simulink model "hcm_segway"  (R2017b)
settings: Solver=ode8  StartTime=0.0  StopTime=10  FixedStep=time_step/10  RelTol=1e-3
values from neighbouring files (symbols this model uses):
  front_rear = 0    [init.m]
  setV = 0    [init.m]
  your_dut = 18    [init.m]
undefined symbols (not defined in the file or in its folder): hcm, sigbuilder_block, Zs0, Zu0
libraries: simulink x2
settings Model: Creator=rvorster  LastModifiedBy=rvorster
settings CodeAppCC: StateflowObjectComments=on
settings SimscapeCC: SimscapeNormalizeSystem=off

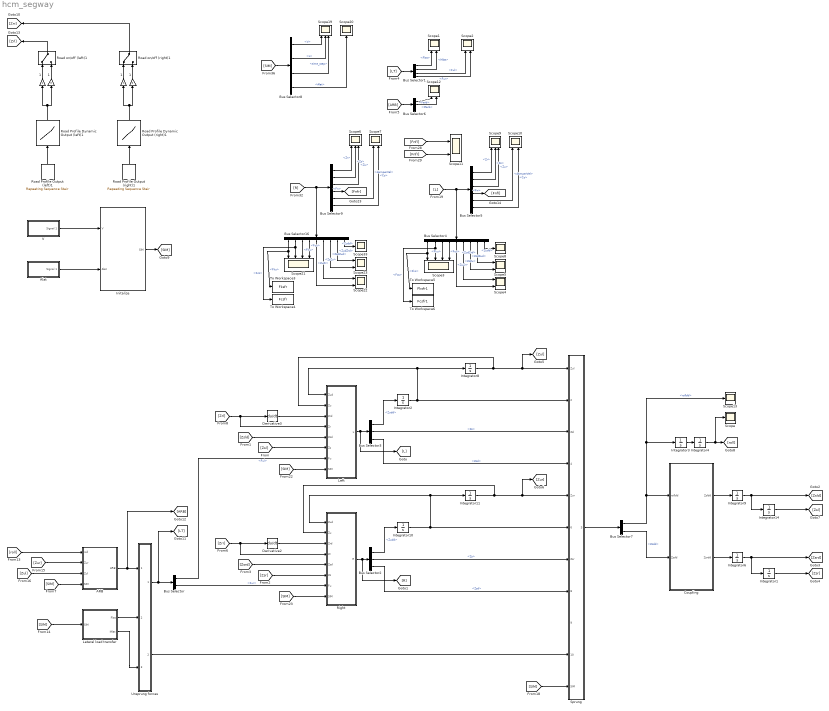
== system hcm_segway ==
  " 1" : Gain  Gain=0
  " 1" : Gain  Gain=0
  " 1" : Gain
  " 1" : Gain
  "ARB " : MATLAB Function  TreatAsAtomicUnit=on
  Alat : Subsystem  Tag=STV Subsys  LoadFcn=sigbuilder_block('load');  StartFcn=sigbuilder_block('start');  StopFcn=sigbuilder_block('stop');  ClipboardFcn=sigbuilder_block('clipboard');  mask(Sigbuilder block){tuvar=[0:10]}
      mask help: Simulink:masks:SigbuilderBlock_MD
      mask init:
      | if ~strcmp(get_param(bdroot(gcbh),'SimulationStatus'),'stopped') tuvar = sigbuilder_block('maskInit'); end
      settings: CopyFcn=sigbuilder_block('copy');  DeleteFcn=sigbuilder_block('delete');  ModelCloseFcn=sigbuilder_block('modelClose');  PreSaveFcn=sigbuilder_block('preSave');  PauseFcn=sigbuilder_block('pause');  ContinueFcn=sigbuilder_block('continue');  NameChangeFcn=sigbuilder_block('namechange');  OpenFcn=sigbuilder_block('open',[429.75 192 565.5 402.75 ]);  CloseFcn=sigbuilder_block('close');
      mask Display: plot(0, 0, 100, 100,[2, 2, 32, 32, 2], [68, 8, 8, 68, 68],[32, 2], [38, 38], [32, 19, 2],[53, 60, 44], [32, 17, 17, 2],[16, 16, 31, 31]);txt = getActiveGroup(gcbh);text(2, 100, txt,'verticalAlignment', 'top');
  Bus Selector : BusSelector  OutputSignals=Ful,Fur
  Bus Selector1 : BusSelector  OutputSignals=Flat,Mlat,Ful,Fur
  Bus Selector16 : BusSelector  OutputSignals=Fks,Fcs,Fku,Fcu,ZuZr,ZsZu,ZsdZud,ZudZrd,Zudd
  Bus Selector2 : BusSelector  OutputSignals=Zudd,Zs,Zsd
  Bus Selector3 : BusSelector  OutputSignals=Zudd,Zs,Zsd
  Bus Selector4 : BusSelector  OutputSignals=Fks,Fcs,Fku,Fcu,ZuZr,ZsZu,ZsdZud,ZudZrd,Zudd
  Bus Selector5 : BusSelector  OutputSignals=Zr,Zs,Zu,Fn,damperVel,Cs
  Bus Selector6 : BusSelector  OutputSignals=Farb,Marb,roll_u
  Bus Selector7 : BusSelector  OutputSignals=rolldd,Zsdd
  Bus Selector8 : BusSelector  OutputSignals=V,L,time_step,Alat
  Bus Selector9 : BusSelector  OutputSignals=Zr,Zs,Zu,Fn,damperVel,Cs
  Coupling : MATLAB Function  TreatAsAtomicUnit=on
  Derivative2 : Derivative
  Derivative3 : Derivative
  Initalize : MATLAB Function  TreatAsAtomicUnit=on
  Integrator1 : Integrator  InitialCondition=-Zs0(2)
  Integrator{2..4,6,9..10} (6 alike) : Integrator
  Integrator11 : Integrator  InitialCondition=-Zu0(2)
  Integrator14 : Integrator  InitialCondition=-Zs0(1)
  Integrator8 : Integrator  InitialCondition=-Zu0(1)
  Lateral load transfer : MATLAB Function  TreatAsAtomicUnit=on
  Left : MATLAB Function  TreatAsAtomicUnit=on
  Right : MATLAB Function  TreatAsAtomicUnit=on
  Road Profile Dynamic Output (left)1 : Lookup_n-D  NumberOfTableDimensions=1  BreakpointsForDimension1=[-5:5]  Table=tanh([-5:5])  InternalRulePriority=Speed  RndMeth=Simplest  InputSameDT=on
  Road Profile Dynamic Output (right)1 : Lookup_n-D  NumberOfTableDimensions=1  BreakpointsForDimension1=[-5:5]  Table=tanh([-5:5])  InternalRulePriority=Speed  RndMeth=Simplest  InputSameDT=on
  Road Profile Output (left)1 : simulink/Sources/Repeating Sequence Stair  OutValues=hx_left  tsamp=time_step  OutMin=[]  OutMax=[]  OutDataTypeStr=double  OutputDataTypeScalingMode=double  OutDataType=fixdt(0,8)  ConRadixGroup=Best Precision: Vector-wise  OutScaling=2^-12
  Road Profile Output (right)1 : simulink/Sources/Repeating Sequence Stair  OutValues=hx_right  tsamp=time_step  OutMin=[]  OutMax=[]  OutDataTypeStr=double  OutputDataTypeScalingMode=double  OutDataType=fixdt(0,8)  ConRadixGroup=Best Precision: Vector-wise  OutScaling=2^-12
  Road on/off (left)1 : ManualSwitch
  Road on/off (right)1 : ManualSwitch
  Scope{,8,13,20,33} (5 alike) : Scope
  Scope{1..2,4..5,7,10..12,22..23} (10 alike) : Scope  NumInputPorts=2
  Scope19 : Scope  NumInputPorts=3
  Scope21 : Scope  NumInputPorts=4
  Scope3 : Scope  NumInputPorts=4
  Scope6 : Scope  NumInputPorts=3
  Scope9 : Scope  NumInputPorts=3
  Sprung : MATLAB Function  TreatAsAtomicUnit=on
  To Workspace3 : ToWorkspace  VariableName=Fksfr  SaveFormat=Timeseries  SampleTime=-1
  To Workspace4 : ToWorkspace  VariableName=Fcsfr  SaveFormat=Timeseries  SampleTime=-1
  To Workspace5 : ToWorkspace  VariableName=Fksfr1  SaveFormat=Timeseries  SampleTime=-1
  To Workspace6 : ToWorkspace  VariableName=Fcsfr1  SaveFormat=Timeseries  SampleTime=-1
  Unsprung forces : MATLAB Function  TreatAsAtomicUnit=on
  V : Subsystem  Tag=STV Subsys  LoadFcn=sigbuilder_block('load');  StartFcn=sigbuilder_block('start');  StopFcn=sigbuilder_block('stop');  ClipboardFcn=sigbuilder_block('clipboard');  mask(Sigbuilder block){tuvar=[0:10]}
      mask help: Simulink:masks:SigbuilderBlock_MD
      mask init:
      | if ~strcmp(get_param(bdroot(gcbh),'SimulationStatus'),'stopped') tuvar = sigbuilder_block('maskInit'); end
      settings: CopyFcn=sigbuilder_block('copy');  DeleteFcn=sigbuilder_block('delete');  ModelCloseFcn=sigbuilder_block('modelClose');  PreSaveFcn=sigbuilder_block('preSave');  PauseFcn=sigbuilder_block('pause');  ContinueFcn=sigbuilder_block('continue');  NameChangeFcn=sigbuilder_block('namechange');  OpenFcn=sigbuilder_block('open',[433.5 195.75 558 401.25 ]);  CloseFcn=sigbuilder_block('close');
      mask Display: plot(0, 0, 100, 100,[2, 2, 32, 32, 2], [68, 8, 8, 68, 68],[32, 2], [38, 38], [32, 19, 2],[53, 60, 44], [32, 17, 17, 2],[16, 16, 31, 31]);txt = getActiveGroup(gcbh);text(2, 100, txt,'verticalAlignment', 'top');
  wires:
  Integrator2/1 -> Sprung/2(Zuld), Left/1(Zud), Integrator8/1
  Left/1(L) -> [L], Bus Selector3/1
  Right/1(R) -> [R], Bus Selector2/1
  Derivative2/1 -> Right/3(Zrd)
  [Zrl] -> Left/4(Zr), Derivative3/1
  [Zrr] -> Right/4(Zr), Derivative2/1
  Bus Selector3/1 -> Integrator2/1  "<Zudd>"
  Derivative3/1 -> Left/3(Zrd)
  [SIM] -> Left/8(SIM)
  Integrator10/1 -> Right/1(Zud), Integrator11/1, Sprung/6(Zurd)
  Integrator11/1 -> Right/2(Zu), Sprung/5(Zur), [Zur]
  [SIM] -> Right/8(SIM)
  Bus Selector2/1 -> Integrator10/1  "<Zudd>"
  Integrator8/1 -> Left/2(Zu), Sprung/1(Zul), [Zul]
  "ARB "/1(ARB) -> Unsprung forces/1(ARB), [ARB]
  [Zul] -> "ARB "/3(Zul)
  [roll] -> "ARB "/1(roll)
  [Zur] -> "ARB "/2(Zur)
  Lateral load transfer/1(Flat) -> Unsprung forces/2(Flat)
  Lateral load transfer/2(Mlat) -> Unsprung forces/3(Mlat)
  [SIM] -> Lateral load transfer/1(SIM)
  Unsprung forces/2(Marbf) -> Sprung/10(Marbf)
  [SIM] -> Sprung/11(SIM)
  " 1"/1 -> Road on/off (left)1/1
  V/1(Signal 1) -> Initalize/1(V)
  " 1"/1 -> Road on/off (right)1/1
  Alat/1(Signal 1) -> Initalize/2(Alat)
  " 1"/1 -> Road on/off (left)1/2
  Road on/off (left)1/1 -> [Zrl]
  Initalize/1(SIM) -> [SIM]
  Road Profile Output (left)1/1 -> Road Profile Dynamic Output (left)1/1
  Road Profile Dynamic Output (left)1/1 -> " 1"/1, " 1"/1
  " 1"/1 -> Road on/off (right)1/2
  Road Profile Dynamic Output (right)1/1 -> " 1"/1, " 1"/1
  Road Profile Output (right)1/1 -> Road Profile Dynamic Output (right)1/1
  Road on/off (right)1/1 -> [Zrr]
  Bus Selector9/3 -> Scope6/3  "<Zu>"
  Bus Selector9/4 -> [Fnfr]  "<Fn>"
  Bus Selector16/2 -> To Workspace4/1, Scope21/2  "<Fcs>"
  Bus Selector16/8 -> Scope23/1  "<ZudZrd>"
  Bus Selector16/3 -> Scope21/3  "<Fku>"
  Bus Selector9/5 -> Scope7/1  "<damperVel>"
  Bus Selector16/4 -> Scope21/4  "<Fcu>"
  Bus Selector16/7 -> Scope23/2  "<ZsdZud>"
  Bus Selector16/6 -> Scope22/1  "<ZsZu>"
  Bus Selector16/5 -> Scope22/2  "<ZuZr>"
  Bus Selector9/6 -> Scope7/2  "<Cs>"
  Bus Selector16/1 -> To Workspace3/1, Scope21/1  "<Fks>"
  [R] -> Bus Selector9/1, Bus Selector16/1
  Bus Selector9/1 -> Scope6/1  "<Zr>"
  Bus Selector9/2 -> Scope6/2  "<Zs>"
  Bus Selector16/9 -> Scope33/1  "<Zudd>"
  Bus Selector4/9 -> Scope8/1  "<Zudd>"
  Bus Selector4/1 -> To Workspace5/1, Scope3/1  "<Fks>"
  [L] -> Bus Selector5/1, Bus Selector4/1
  Bus Selector5/2 -> Scope9/2  "<Zs>"
  Bus Selector5/6 -> Scope10/2  "<Cs>"
  Bus Selector4/6 -> Scope4/1  "<ZsZu>"
  Bus Selector4/7 -> Scope5/2  "<ZsdZud>"
  Bus Selector4/4 -> Scope3/4  "<Fcu>"
  Bus Selector4/3 -> Scope3/3  "<Fku>"
  Bus Selector5/1 -> Scope9/1  "<Zr>"
  Bus Selector4/5 -> Scope4/2  "<ZuZr>"
  Bus Selector5/4 -> [Fnfl]  "<Fn>"
  Bus Selector5/5 -> Scope10/1  "<damperVel>"
  Bus Selector4/2 -> To Workspace6/1, Scope3/2  "<Fcs>"
  Bus Selector5/3 -> Scope9/3  "<Zu>"
  Bus Selector4/8 -> Scope5/1  "<ZudZrd>"
  [Fnfl] -> Scope11/1
  [Fnfr] -> Scope11/2
  Bus Selector8/4 -> Scope20/1  "<Alat>"
  Bus Selector8/2 -> Scope19/2  "<L>"
  [SIM] -> Bus Selector8/1
  Bus Selector8/1 -> Scope19/1  "<V>"
  Bus Selector8/3 -> Scope19/3  "<time_step>"
  Bus Selector3/2 -> Sprung/3(Zsl)  "<Zs>"
  Bus Selector3/3 -> Sprung/4(Zsld)  "<Zsd>"
  Bus Selector2/2 -> Sprung/7(Zsr)  "<Zs>"
  Bus Selector2/3 -> Sprung/8(Zsrd)  "<Zsd>"
  Sprung/1(S) -> Bus Selector7/1
  Coupling/1(Zsldd) -> Integrator9/1
  Integrator9/1 -> [Zsld], Integrator14/1
  Coupling/2(Zsrdd) -> Integrator6/1
  Integrator6/1 -> [Zsrd], Integrator1/1
  Integrator1/1 -> [Zsr]
  Integrator14/1 -> [Zsl]
  [Zsl] -> Left/6(Zs)
  [Zsld] -> Left/5(Zsd)
  [Zsrd] -> Right/5(Zsd)
  [Zsr] -> Right/6(Zs)
  Integrator3/1 -> Integrator4/1
  Integrator4/1 -> Scope/1, [roll]
  Unsprung forces/1(LT) -> [LT], Bus Selector/1
  Bus Selector/1 -> Left/7(Fu)  "<Ful>"
  Bus Selector/2 -> Right/7(Fu)  "<Fur>"
  [LT] -> Bus Selector1/1
  Bus Selector1/1 -> Scope1/1  "<Flat>"
  Bus Selector1/2 -> Scope1/2  "<Mlat>"
  Bus Selector1/3 -> Scope2/1  "<Ful>"
  Bus Selector1/4 -> Scope2/2  "<Fur>"
  [ARB] -> Bus Selector6/1
  Bus Selector6/1 -> Scope12/1  "<Farb>"
  Bus Selector6/2 -> Scope12/2  "<Marb>"
  Bus Selector7/1 -> Coupling/1(rolldd), Scope13/1, Integrator3/1  "<rolldd>"
  Bus Selector7/2 -> Coupling/2(Zsdd)  "<Zsdd>"
  [SIM] -> "ARB "/4(SIM)

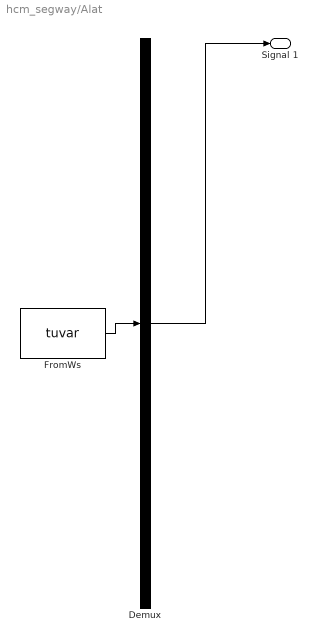
== system hcm_segway/Alat ==
  Demux : Demux  Tag=STV Demux  Outputs=1
  FromWs : FromWorkspace  Tag=STV FromWs  VariableName=tuvar  SampleTime=0
      SigBuilderData=|
      | common.afterFinalStr = 'Extrapolate'
      | common.sampleTime = 0
      | dataSet.timeRange = [0 10]
      | dataSet.name = 'Group 1'
      | sbobj.Groups.Name = 'Group 1'
      | sbobj.Groups.Signals.Name = 'Signal 1'
      | sbobj.Groups.Signals.XData = [0 4 6 10]
      | sbobj.Groups.Signals.YData = [0 0 0 0]
  Signal 1 : Outport  Tag=STV Outport
  wires:
  Demux/1 -> Signal 1/1
  FromWs/1 -> Demux/1

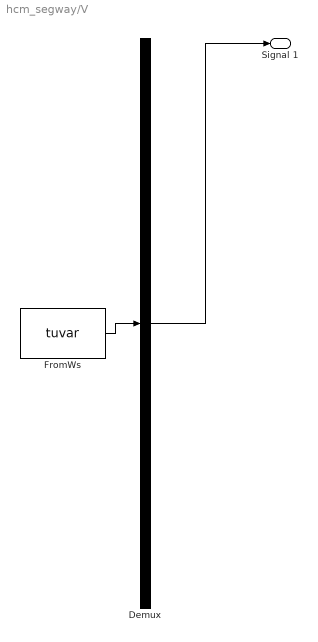
== system hcm_segway/V ==
  Demux : Demux  Tag=STV Demux  Outputs=1
  FromWs : FromWorkspace  Tag=STV FromWs  VariableName=tuvar  SampleTime=0
      SigBuilderData=|
      | common.afterFinalStr = 'Extrapolate'
      | common.sampleTime = 0
      | dataSet.timeRange = [0 10]
      | dataSet.name = 'Group 1'
      | sbobj.Groups.Name = 'Group 1'
      | sbobj.Groups.Signals.Name = 'Signal 1'
      | sbobj.Groups.Signals.XData = [0 4 6 10]
      | sbobj.Groups.Signals.YData = [0 35 0 0]
  Signal 1 : Outport  Tag=STV Outport
  wires:
  Demux/1 -> Signal 1/1
  FromWs/1 -> Demux/1

== matlab function hcm_segway/Right ==
  data: Zud input; Zu input; Zrd input; Zr input; Zsd input; Zs input; Fu input; hcm parameter; R output Bus: U; SIM input Bus: SIM; Zs0 parameter
function R = fcn(Zud, Zu, Zrd, Zr, Zsd, Zs, Fu, hcm, SIM, Zs0)
    
    loc = 1;
    R = unsprung_mass(Zud, Zu, Zrd, Zr, Zsd, Zs, Fu, loc, SIM, Zs0, hcm);

end

== matlab function hcm_segway/Left ==
  data: Zud input; Zu input; Zrd input; Zr input; Zsd input; Zs input; Fu input; hcm parameter; L output Bus: U; SIM input Bus: SIM; Zs0 parameter
function L = fcn(Zud, Zu, Zrd, Zr, Zsd, Zs, Fu, hcm, SIM, Zs0)

    if (SIM.front_rear == 0)
        loc = 1;
    else
        loc = 3;
    end

    L = unsprung_mass(Zud, Zu, Zrd, Zr, Zsd, Zs, Fu, loc, SIM, Zs0, hcm);

end

== matlab function hcm_segway/Sprung ==
  data: Zul input; Zuld input; S output Bus: C; Zsl input; Zsld input; Zur input; Zurd input; Zsr input; Zsrd input; Mlatf input; Marbf input; SIM input Bus: SIM; hcm parameter
function S = fcn(Zul, Zuld, Zsl, Zsld, Zur, Zurd, Zsr, Zsrd, Mlatf, Marbf, SIM, hcm)   
    
    S = sprung_mass_segway(Zul, Zuld, Zsl, Zsld, Zur, Zurd, Zsr, ... 
        Zsrd, Mlatf, Marbf, SIM, hcm);

end

== matlab function hcm_segway/ARB  ==
  settings: updateMethod=DISCRETE
  data: roll input; Zur input; Zul input; SIM input Bus: SIM; hcm parameter; ARB output Bus: ARB
function ARB = fcn(roll, Zur, Zul, SIM, hcm)

    ARB = arb(Zur, Zul, roll, SIM, hcm);
    
end

== matlab function hcm_segway/Unsprung forces ==
  data: LT output Bus: LT; ARB input; Flat input; Mlat input; Marbf output
function [LT, Marbf] = fcn(ARB, Flat, Mlat)
    
    Marbf = ARB.Marb;
    
    LT.Flat = Flat;
    LT.Mlat = Mlat;
    LT.Flongf = 0;
    LT.Flongr = 0;
    LT.Mlong = 0;
    
    LT.Ful = -(ARB.Farb + Flat);
    LT.Fur = ARB.Farb + Flat;
    
end

== matlab function hcm_segway/Lateral load transfer ==
  data: Flat output; Mlat output; hcm parameter; SIM input Bus: SIM
function [Flat, Mlat] = fcn(hcm, SIM)
    
    [Flat, Mlat] = lateral_load(SIM, hcm);
    
end

== matlab function hcm_segway/Coupling ==
  data: rolldd input; Zsldd output; Zsrdd output; Zsdd input; hcm parameter
function [Zsldd, Zsrdd] = fcn(rolldd, Zsdd, hcm)

    [Zsldd, Zsrdd] = coupling_segway(Zsdd, rolldd, hcm);

end

== matlab function hcm_segway/Initalize ==
  settings: updateMethod=DISCRETE
  data: V input; Alat input; hcm parameter; SIM output Bus: SIM; setV parameter; front_rear parameter; your_dut parameter
function SIM = fcn(V, Alat, hcm, setV, front_rear, your_dut)

    if (setV == 0)
        SIM.V = hcm.V;
        SIM.L = 0.5*hcm.V^2*hcm.ClA*hcm.rho0;
        SIM.Alat = hcm.Alat;
        SIM.Along = 0;
        SIM.sim_time = 0;
        SIM.sim_step = 0;
        SIM.time_step = 0.01 / hcm.V;
        SIM.your_dut = your_dut;
        SIM.front_rear = front_rear;
    else
        SIM.V = V;
        SIM.L = 0.5*V^2*hcm.ClA*hcm.rho0;
        SIM.Alat = Alat;
        SIM.Along = 0;
        SIM.sim_time = 0;
        SIM.sim_step = 0;
        SIM.time_step = 0.01 / V;
        SIM.your_dut = your_dut;
        SIM.front_rear = front_rear;
    end

end
